simulink model "Calculate"  (R2018b)
settings: Solver=FixedStepDiscrete  StartTime=0.0  StopTime=10.0  RelTol=1e-3
settings Model: Creator=matlab  LastModifiedBy=matlab
settings DataIOCC: SaveOutput=off  SignalLogging=off  SaveTime=off
settings OptimizationCC: DefaultParameterBehavior=Inlined  EnhancedBackFolding=on  PassReuseOutputArgsAs=Individual arguments  OptimizeBlockOrder=speed  DifferentSizesBufferReuse=on  OptimizationCustomize=off
settings DebuggingCC: ParameterTunabilityLossMsg=error
settings SFSimCC: MATLABDynamicMemAlloc=off
settings RTWCC: SystemTargetFile=ert.tlc  TemplateMakefile=ert_default_tmf  PostCodeGenCommand=packNGo(buildInfo);  GenerateReport=on  IncludeHyperlinkInReport=on  LaunchReport=on  GenerateTraceInfo=on  GenerateTraceReport=on  GenerateTraceReportSl=on  GenerateTraceReportSf=on  GenerateTraceReportEml=on
settings CodeAppCC: ForceParamTrailComments=on  IgnoreCustomStorageClasses=off  OperatorAnnotations=on  SimulinkDataObjDesc=on  SFDataObjDesc=on  InsertBlockDesc=on
settings ERTTargetCC: TargetLangStandard=C99 (ISO)  GenerateSampleERTMain=on  InlinedParameterPlacement=NonHierarchical  ERTCustomFileTemplate=example_file_process.tlc

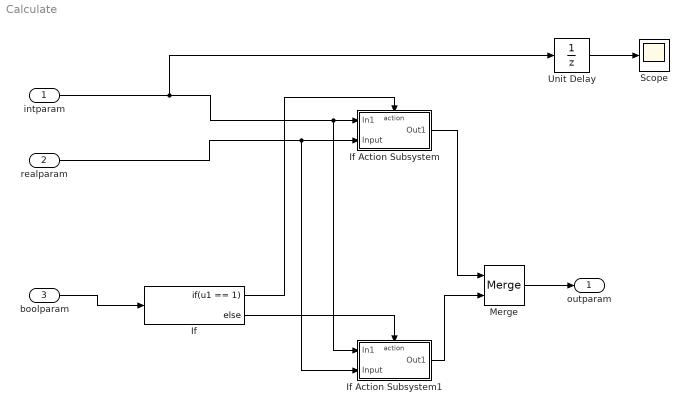
== system Calculate ==
  intparam : Inport  OutDataTypeStr=MyInteger  BusOutputAsStruct=on
  realparam : Inport  Port=2  OutDataTypeStr=MyReal  BusOutputAsStruct=on
  boolparam : Inport  Port=3  OutDataTypeStr=MyBool  BusOutputAsStruct=on
  If : If  IfExpression=u1 == 1
  If Action Subsystem : Subsystem  TreatAsAtomicUnit=on
  If Action Subsystem1 : Subsystem  TreatAsAtomicUnit=on
  Merge : Merge
  Scope : Scope
  Unit Delay : UnitDelay  SampleTime=-1
  outparam : Outport  OutDataTypeStr=MyReal
  wires:
  boolparam/1 -> If/1
  If/1 -> If Action Subsystem/Action
  intparam/1 -> Unit Delay/1, If Action Subsystem1/1(In1), If Action Subsystem/1(In1)
  realparam/1 -> If Action Subsystem1/2(Input), If Action Subsystem/2(Input)
  Merge/1 -> outparam/1
  If Action Subsystem/1(Out1) -> Merge/1
  If Action Subsystem1/1(Out1) -> Merge/2
  If/2 -> If Action Subsystem1/Action
  Unit Delay/1 -> Scope/1

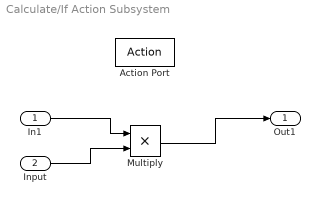
== system Calculate/If Action Subsystem ==
  In1 : Inport
  Input : Inport  Port=2
  Action Port : ActionPort  ActionType=then
  Multiply : Product
  Out1 : Outport
  wires:
  Input/1 -> Multiply/2
  In1/1 -> Multiply/1
  Multiply/1 -> Out1/1

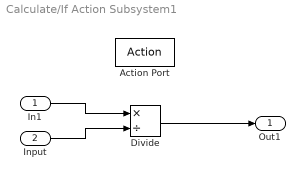
== system Calculate/If Action Subsystem1 ==
  In1 : Inport
  Input : Inport  Port=2
  Action Port : ActionPort  ActionType=else
  Divide : Product  Inputs=*/
  Out1 : Outport
  wires:
  In1/1 -> Divide/1
  Divide/1 -> Out1/1
  Input/1 -> Divide/2
